simulink model "Q2"  (R2020b)
settings: Solver=VariableStepAuto  StartTime=0.0  StopTime=10.0  RelTol=1e-3
libraries: simulink x1
settings Model: Creator=Lenovo  LastModifiedBy=Lenovo

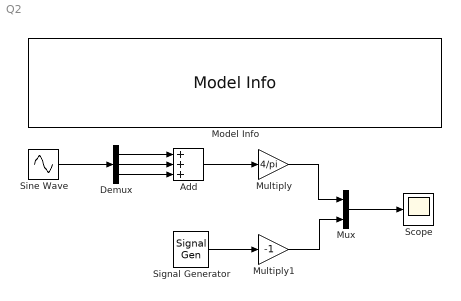
== system Q2 ==
  Add : Sum  Inputs=+++
  Demux : Demux  Outputs=3
  Model Info : simulink/Model-Wide Utilities/Model Info  Frame=on  DisplayStringWithTags=|  HorizontalTextAlignment=Center  LeftAlignmentValue=0.5
      | EE520 Q1.2  Furkan Sönmez
      | 
      | Simulink Model for Summation of 3 different Signal Waves with constant multiplier( i.e. 4/pi )
      |  Amp = [1 1/3 1/5] Volt
      |  Freq = [1 3 5 ] rad/sec
      |  Phase= [0 0 0 ] rad
      | Sample Time =0.01
      | Simulation duration= 10 sec
  Multiply : Gain  Gain=4/pi
  Multiply1 : Gain  Gain=-1
  Mux : Mux  Inputs=2
  Scope : Scope
  Signal Generator : SignalGenerator  WaveForm=square  Units=rad/sec
  Sine Wave : Sin  Amplitude=[1 1/3 1/5]  Bias=[0 0 0]  Frequency=[1 3 5]  Phase=[0 0 0]  SampleTime=0.01
  wires:
  Sine Wave/1 -> Demux/1
  Demux/1 -> Add/1
  Demux/2 -> Add/2
  Demux/3 -> Add/3
  Add/1 -> Multiply/1
  Signal Generator/1 -> Multiply1/1
  Multiply/1 -> Mux/1
  Multiply1/1 -> Mux/2
  Mux/1 -> Scope/1
